simulink model "dspstfft_win32"  (Simulink 6.0)
settings: Solver=FixedStepDiscrete  StartTime=0.0  StopTime=inf  RelTol=1e-3
undefined symbols (not defined in the file or in its folder): jet
libraries: dspbuff3 x2, dspsnks4 x2, dspwin32 x1, dspspect3 x1, dspmtrx3 x1, dspmathops x1
settings Model: Creator=jeff  LastModifiedBy=hzarrink  SaveTime=off  SaveOutput=off  SignalLoggingName=logsOut  BlockReductionOpt=off  ZeroCrossControl=UseLocalSettings  ProdHWDeviceType=Microprocessor  TargetHWChar=2  TargetHWWordLengths=8,16,32,32  RTWMathFcnLibMatFile=iso_c_tmw.mat  RTWOptions="-aEnforceIntegerDowncast=1 -aFoldNonRolledExpr=1 -aInlineInvariantSignals=1 -aInlineParameters=0 -aLocalBlockOutputs=1 -aRollThreshold=5 -aGenerateReport=0 -aGenCodeOnly=0 -aRTWVerbose=1 -aForceParamTrailComments=0 -aGenerateComments=1 -aIgnoreCustomStorageClasses=1 -aIncHierarchyInIds=0 -aMaxRTWIdLen=31 -aShowEliminatedStatements=0 -aPrefixModelToSubsysFcnNames=1 -aIncDataTypeInIds=0 -aInlinedPrmAccess=\"Literals\" -aTargetFcnLib=\"iso_c_tmw.mat\" -aGenerateFullHeader=1 -aIsPILTarget=0 -aExtMode=0 -aExtModeStaticAlloc=0 -aExtModeTesting=0 -aExtModeStaticAllocSize=1000000 -aExtModeTransport=0 -aLogVarNameModifier=\"rt_\" -aRTWCAPISignals=0 -aRTWCAPIParams=0"
settings DataIOCC: SaveOutput=off  SaveTime=off  SignalLoggingName=logsOut
settings OptimizationCC: BlockReduction=off  BooleanDataType=off  MultiInstanced=off
settings FormatCC: IgnoreBidirectionalLines=off
settings HardwareCC: ProdHWDeviceType=Microprocessor  ShiftRightIntArith=on  TargetHWCharacteristics=InheritFromRTWHook
settings CodeAppCC: FileBanners=off
settings GRTTargetCC: TargetFcnLib=iso_c_tmw.mat  IsERTTarget=off

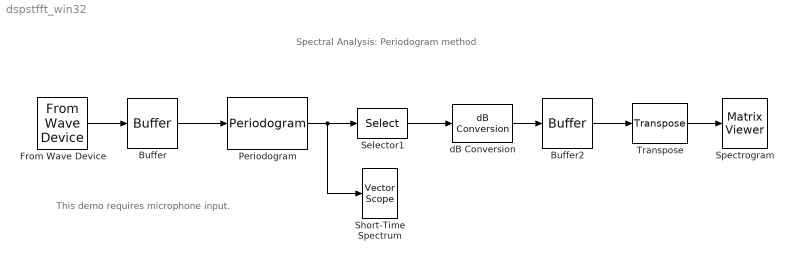
== system dspstfft_win32 ==
  note: This demo requires microphone input.
  note: Spectral Analysis: Periodogram method
  Buffer : dspbuff3/Buffer  N=128  V=48  ic=0
  Buffer2 : dspbuff3/Buffer  N=48  V=46  ic=-70
  From Wave Device : dspwin32/From Wave Device  SampleRate=8000  UserRate=16000  SampleWidth=16  Stereo=off  SamplesPerFrame=256  QueueDuration=1  useDefaultDevice=on  dType=double
  Periodogram : dspspect3/Periodogram  wintype=Hamming  Rs=50  beta=5  winsamp=Periodic  inheritFFT=on  fftsize=128  navg=2
  Selector1 : Selector  Elements=1:64  InputPortWidth=128
  Short-Time Spectrum : dspsnks4/Vector Scope  ScopeProperties=on  Domain=Frequency  HorizSpan=1  DisplayProperties=off  AxisGrid=off  Memory=off  FrameNumber=off  AxisLegend=off  AxisZoom=off  OpenScopeAtSimStart=on  OpenScopeImmediately=off  FigPos=[80 110 380 320]  AxisProperties=off  XUnits=Hertz  XRange=[0...Fs/2]  InheritXIncr=on  XIncr=1  XLabel=Samples  YUnits=dB  YLabel=Magnitude, dB  LineProperties=off
      settings: YMin=-59.7576717829863  YMax=9.71199466608513
  Spectrogram : dspsnks4/Matrix Viewer  ImageParams=off  CMapStr=jet(256)  AxisColorbar=on  AxisParams=off  AxisOrigin=Lower left corner  XLabel=Time Index  YLabel=Frequency Index  ZLabel=dB Magnitude  FigPos=[468 110 380 320]  AxisZoom=off
      settings: YMin=-70  YMax=15
  Transpose : dspmtrx3/Transpose  Hermitian=off
  dB Conversion : dspmathops/dB Conversion  dBtype=dB  intype=Amplitude  R=1  fuzz=on
  wires:
  Buffer/1 -> Periodogram/1
  From Wave Device/1 -> Buffer/1
  Selector1/1 -> dB Conversion/1
  dB Conversion/1 -> Buffer2/1
  Buffer2/1 -> Transpose/1
  Transpose/1 -> Spectrogram/1
  Periodogram/1 -> Selector1/1, Short-Time Spectrum/1
